simulink model "hcs"  (Simulink 8.3)
settings: Solver=ode45  StartTime=0.0  StopTime=10  RelTol=1e-10
settings Model: Creator=liang  LastModifiedBy=yangg
settings DataIOCC: MaxDataPoints=10000000  SaveFormat=StructureWithTime
settings OptimizationCC: ExpressionDepthLimit=2147483647
settings DebuggingCC: FcnCallInpInsideContextMsg=EnableAllAsWarning
settings GRTTargetCC: CombineOutputUpdateFcns=on  GRTInterface=off

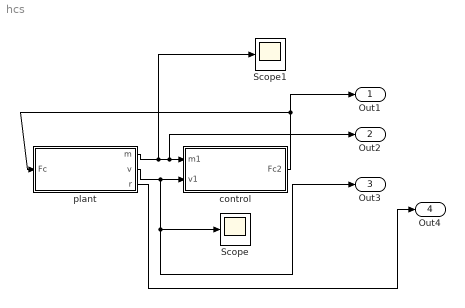
== system hcs ==
  Scope : Scope
      settings: YMin=-2  YMax=-1.9998
  Scope1 : Scope
      settings: TimeRange=100  YMin=-2  YMax=-1.9998  SaveName=ScopeData2
  control : Subsystem
  plant : Subsystem
  Out1 : Outport
  Out2 : Outport  Port=2
  Out3 : Outport  Port=3
  Out4 : Outport  Port=4
  wires:
  plant/1(m) -> Scope1/1, Out2/1, control/1(m1)
  plant/2(v) -> Out3/1, Scope/1, control/2(v1)
  control/1(Fc2) -> plant/1(Fc), Out1/1
  plant/3(r) -> Out4/1

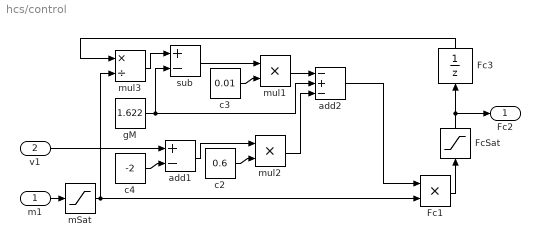
== system hcs/control ==
  m1 : Inport
  v1 : Inport  Port=2
  Fc1 : Product  Inputs=**  SampleTime=0.128
  Fc3 : UnitDelay  InitialCondition=2027.5  SampleTime=-1
  FcSat : Saturate  UpperLimit=5000  LowerLimit=1500  SampleTime=0.128
  add1 : Sum  Inputs=+-  SampleTime=0.128
  add2 : Sum  Inputs=-+-  SampleTime=0.128
  c2 : Constant  Value=0.6
  c3 : Constant  Value=0.01
  c4 : Constant  Value=-2
  gM : Constant  Value=1.622
  mSat : Saturate  UpperLimit=3000  LowerLimit=1100  SampleTime=0.128
  mul1 : Product  Inputs=**  SampleTime=0.128
  mul2 : Product  Inputs=**  SampleTime=0.128
  mul3 : Product  Inputs=*/  SampleTime=0.128
  sub : Sum  Inputs=+-  SampleTime=0.128
  Fc2 : Outport
  wires:
  m1/1 -> mSat/1
  mul3/1 -> sub/1
  gM/1 -> add2/2, sub/2
  sub/1 -> mul1/1
  c3/1 -> mul1/2
  c4/1 -> add1/2
  add1/1 -> mul2/1
  c2/1 -> mul2/2
  mul2/1 -> add2/3
  v1/1 -> add1/1
  Fc1/1 -> FcSat/1
  Fc3/1 -> mul3/1
  mul1/1 -> add2/1
  mSat/1 -> mul3/2, Fc1/2
  FcSat/1 -> Fc3/1, Fc2/1
  add2/1 -> Fc1/1

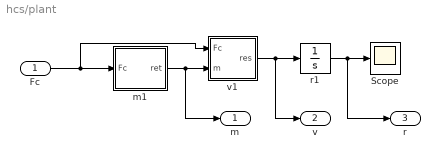
== system hcs/plant ==
  Fc : Inport
  Scope : Scope
      settings: TimeRange=14  YMin=5.85  YMax=6.22
  m1 : Subsystem
  r1 : Integrator  InitialCondition=30
  v1 : Subsystem
  m : Outport
  v : Outport  Port=2
  r : Outport  Port=3
  wires:
  m1/1(ret) -> v1/2(m), m/1
  v1/1(res) -> v/1, r1/1
  Fc/1 -> v1/1(Fc), m1/1(Fc)
  r1/1 -> r/1, Scope/1

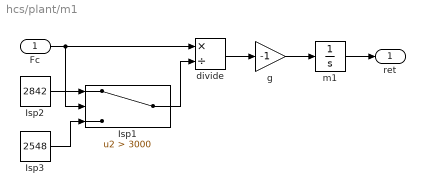
== system hcs/plant/m1 ==
  Fc : Inport
  Isp1 : Switch  Criteria=u2 > Threshold  Threshold=3000  SampleTime=0.001
  Isp2 : Constant  Value=2842
  Isp3 : Constant  Value=2548
  divide : Product  Inputs=*/  SampleTime=0.001
  g : Gain  Gain=-1  SampleTime=0.001
  m1 : Integrator  InitialCondition=1250
  ret : Outport
  wires:
  Fc/1 -> divide/1, Isp1/2
  divide/1 -> g/1
  g/1 -> m1/1
  m1/1 -> ret/1
  Isp2/1 -> Isp1/1
  Isp3/1 -> Isp1/3
  Isp1/1 -> divide/2

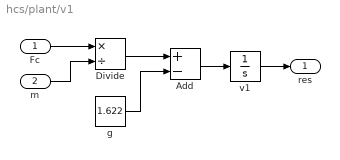
== system hcs/plant/v1 ==
  Fc : Inport
  m : Inport  Port=2
  Add : Sum  Inputs=+-  SampleTime=0.001
  Divide : Product  Inputs=*/  SampleTime=0.001
  g : Constant  Value=1.622
  v1 : Integrator  InitialCondition=-2
  res : Outport
  wires:
  Fc/1 -> Divide/1
  m/1 -> Divide/2
  Divide/1 -> Add/1
  g/1 -> Add/2
  Add/1 -> v1/1
  v1/1 -> res/1
